simulink model "Simulation_Observer"  (R2021a)
settings: Solver=VariableStepAuto  StartTime=ti  StopTime=tf  RelTol=1e-3
undefined symbols (not defined in the file): a, Noise, omega
libraries: simulink x1
settings Model: Creator=perruquetti  LastModifiedBy=perruquetti
settings SolverCC: AlgebraicLoopSolver=TrustRegion
settings DataIOCC: ReturnWorkspaceOutputs=off
settings DebuggingCC: SFMachineParentedDataDiag=warning  ArithmeticOperatorsInVariantConditions=warning
settings SFSimCC: SimUseLocalCustomCode=off  CustomCodeUndefinedFunction=UseInterfaceOnly
settings RTWCC: RTWUseLocalCustomCode=off

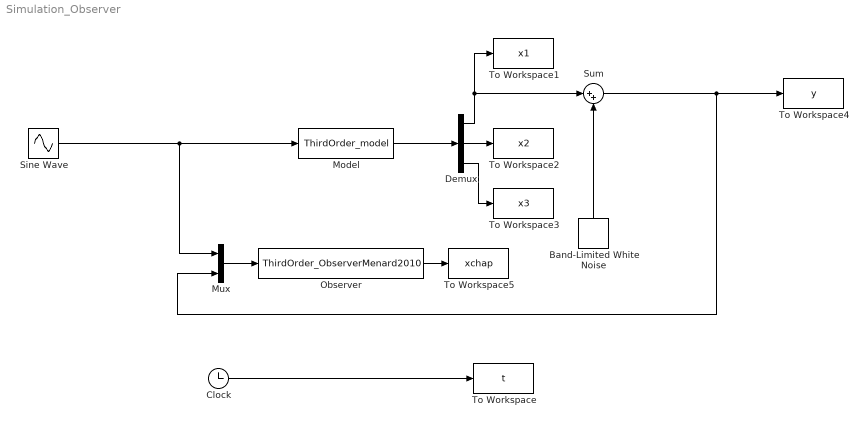
== system Simulation_Observer ==
  Band-Limited White Noise : simulink/Sources/Band-Limited White Noise  Cov=Noise.power  Ts=Noise.sampling  seed=Noise.seed
  Clock : Clock
  Demux : Demux  Outputs=3
  Model : S-Function  FunctionName=ThirdOrder_model  SFunctionDeploymentMode=off  EnableBusSupport=off
  Mux : Mux  Inputs=2
  Observer : S-Function  FunctionName=ThirdOrder_ObserverMenard2010  Parameters=params_observer  SFunctionDeploymentMode=off  EnableBusSupport=off
  Sine Wave : Sin  Amplitude=a  Frequency=omega  SampleTime=0
  Sum : Sum  Inputs=|++
  To Workspace : ToWorkspace  VariableName=t  SampleTime=-1
  To Workspace1 : ToWorkspace  VariableName=x1  SampleTime=-1
  To Workspace2 : ToWorkspace  VariableName=x2  SampleTime=-1
  To Workspace3 : ToWorkspace  VariableName=x3  SampleTime=-1
  To Workspace4 : ToWorkspace  VariableName=y  SampleTime=-1
  To Workspace5 : ToWorkspace  VariableName=xchap  SampleTime=-1
  wires:
  Clock/1 -> To Workspace/1
  Model/1 -> Demux/1
  Band-Limited White Noise/1 -> Sum/2
  Demux/1 -> To Workspace1/1, Sum/1
  Mux/1 -> Observer/1
  Sine Wave/1 -> Mux/1, Model/1
  Sum/1 -> Mux/2, To Workspace4/1
  Demux/2 -> To Workspace2/1
  Observer/1 -> To Workspace5/1
  Demux/3 -> To Workspace3/1
